simulink model "Task4"  (R2024a)
settings: Solver=VariableStepAuto  StartTime=0.0  StopTime=2400.0  RelTol=1e-3
settings Model: Creator=artemzmailov  LastModifiedBy=artemzmailov

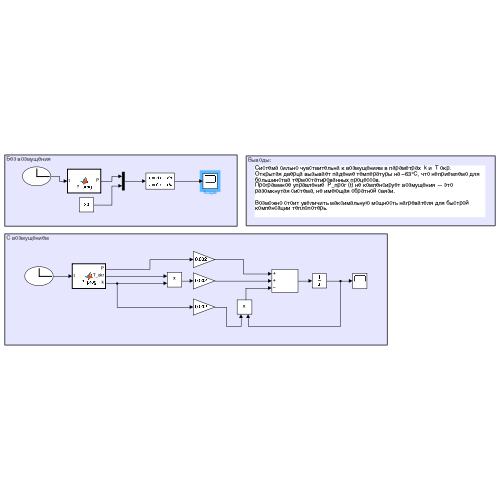
[thumbnail: Simulink's stored preview of the top-level diagram]
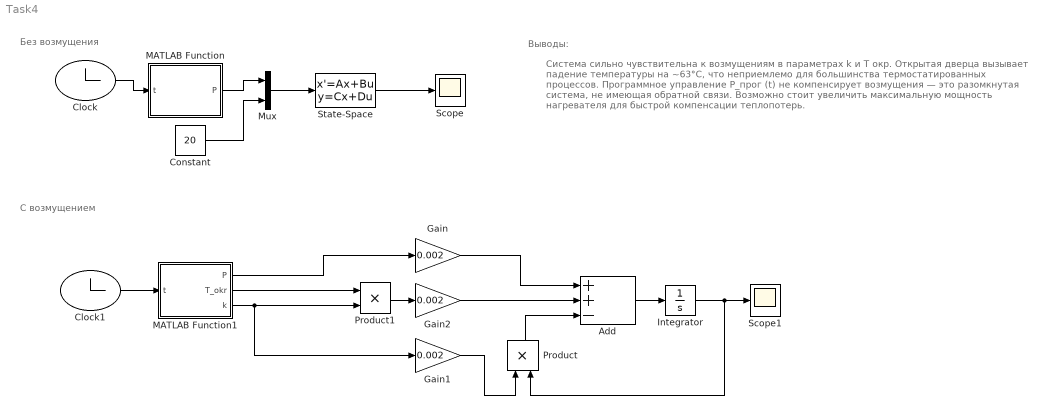
== system Task4 ==
  note: Выводы:
  note: Система сильно чувствительна к возмущениям в параметрах k и T окр.
      | Открытая дверца вызывает падение температуры на ~63°C, что неприемлемо для большинства термостатированных процессов.
      | Программное управление P_прог (t) не компенсирует возмущения — это разомкнутая система, не имеющая обратной связи.
      |
      | Возможно стоит увеличить максимальную мощность нагревателя для быстрой компенсации теплопотерь.
  note: Без возмущения
  note: С возмущением
  Add : Sum  Inputs=++-
  Clock : Clock
  Clock1 : Clock
  Constant : Constant  Value=20
  Gain : Gain  Gain=0.002
  Gain1 : Gain  Gain=0.002
  Gain2 : Gain  Gain=0.002
  Integrator : Integrator  InitialCondition=20
  MATLAB Function : MATLAB Function  TreatAsAtomicUnit=on
  MATLAB Function1 : MATLAB Function  TreatAsAtomicUnit=on
  Mux : Mux  Inputs=2
  Product : Product
  Product1 : Product
  Scope : Scope
  Scope1 : Scope
  State-Space : StateSpace  A=-0.02  B=[0.002, 0.02]  D=[0,0]  InitialCondition=20
  wires:
  Clock/1 -> MATLAB Function/1(t)
  State-Space/1 -> Scope/1
  MATLAB Function/1(P) -> Mux/1
  Constant/1 -> Mux/2
  Mux/1 -> State-Space/1
  Clock1/1 -> MATLAB Function1/1(t)
  MATLAB Function1/1(P) -> Gain/1
  Gain/1 -> Add/1
  Add/1 -> Integrator/1
  MATLAB Function1/3(k) -> Gain1/1, Product1/2
  Integrator/1 -> Product/2, Scope1/1
  Product/1 -> Add/3
  MATLAB Function1/2(T_okr) -> Product1/1
  Product1/1 -> Gain2/1
  Gain2/1 -> Add/2
  Gain1/1 -> Product/1

== matlab function Task4/MATLAB Function1 ==
  data: t input; P output; T_okr output; k output
function [P, T_okr, k] = P_prog(t)
    if t <= 600
        P = 200/3 + (4/3)*t;
    else 
        P = 800;
    end

    if (t < 900) || (t > 1020)
        T_okr = 20;
        k = 10;
    else
        T_okr = 5;
        k = 25;
    end
end

== matlab function Task4/MATLAB Function ==
  data: t input; P output
function P = P_prog(t)
    if t <= 600
        P = 200/3 + (4/3)*t;
    else 
        P = 800;
    end
end
